simulink model "velocidades"  (R2023b)
settings: Solver=ode14x  StartTime=0.0  StopTime=10.0  FixedStep=0.005  RelTol=1e-3
values from neighbouring files (symbols this model uses):
  a = parametros(1)    [erro_velocidades.m]
  b = 0.02    [Teste1_velocidades.m]    (also in erro_velocidades.m = parametros(2))
  K = Vss*b/300    [erro_velocidades.m]
  T = t(129:286,1)-t(129)    [Teste1_velocidades.m]
  VDes = p(129:286,1)    [Teste1_velocidades.m]
  VReal = Vin(129:286,1)    [Teste1_velocidades.m]
libraries: cstblocks x1
settings Model: Creator=alexa  LastModifiedBy=henri

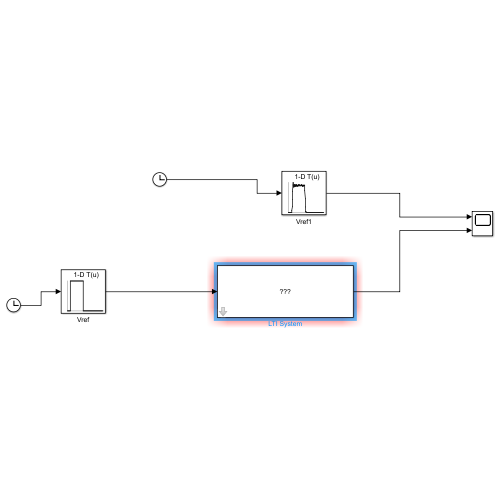
[thumbnail: Simulink's stored preview of the top-level diagram]
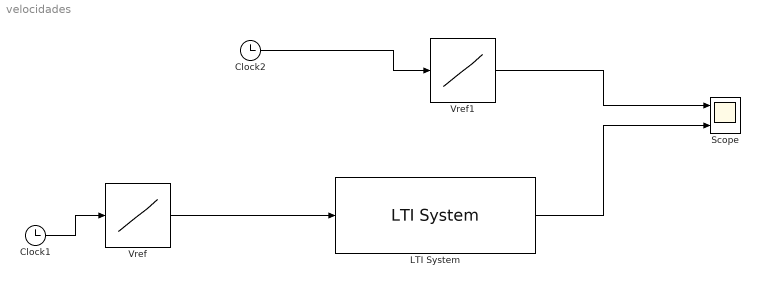
== system velocidades ==
  Clock1 : Clock
  Clock2 : Clock
  LTI System : cstblocks/LTI System  sys=tf(K,[1 a b], 'InputDelay',0.1)  IC=[]  PadeOrder=0
  Scope : Scope  NumInputPorts=2
  Vref : Lookup_n-D  NumberOfTableDimensions=1  BreakpointsForDimension1=T  Table=VDes  InternalRulePriority=Speed  RndMeth=Simplest
  Vref1 : Lookup_n-D  NumberOfTableDimensions=1  BreakpointsForDimension1=T  Table=VReal  InternalRulePriority=Speed  RndMeth=Simplest
  wires:
  Clock1/1 -> Vref/1
  Clock2/1 -> Vref1/1
  Vref1/1 -> Scope/1
  Vref/1 -> LTI System/1
  LTI System/1 -> Scope/2
